simulink model "BD_PRIUS_JPN"  (Simulink 7.9)
settings: Solver=ode1  SolverMode=SingleTasking  StartTime=0.0  StopTime=max(cyc_mph(:,1))  FixedStep=1  MaxStep=1  RelTol=1e-3  AbsTol=1e-3
undefined symbols (not defined in the file): ex_calc, fc_emis
libraries: lib_wheel x2, lib_help x2, lib_transmission x2, lib_electric_machine x2, lib_outputs x1, lib_controls x1, lib_interactive x1, lib_drive_cycle x1, lib_energy_storage x1, lib_exhaust x1, lib_fuel_converter x1, lib_power_bus x1
settings Model: Creator=mokeefe  LastModifiedBy=mokeefe  ExtModeTrigMode=oneshot  ExtModeArmWhenConnect=off
settings Model: ModifiedComment=|
  | mokeefe -- Fri Apr 06 09:40:25 2012 -- Version 1.42
  | Update library links.
settings Model: ModifiedHistory=|
  | mokeefe -- Fri Apr 06 09:40:25 2012 -- Version 1.42
  | Update library links.
  | 
  | mokeefe -- Fri Apr 06 09:31:50 2012 -- Version 1.41
  | Save as latest simulink version.
  | 
  | ssprik -- Wed Sep 24 15:15:04 2003 -- Version 1.40
  | 
  | 
  | abrooker -- Tue May 14 11:47:35 2002 -- Version 1.39
  | 
  | 
  | mokeefe -- Thu Apr 18 08:05:37 2002 -- Version 1.38
  | saving the model:
  | o "without the model browser open"
  | o with only top-level screen visible
  | o and with "fit to view" enabled
settings DataIOCC: LimitDataPoints=off  SaveOutput=off  SaveTime=off
settings OptimizationCC: BooleanDataType=off
settings DebuggingCC: SaveWithParameterizedLinksMsg=none  SignalResolutionControl=TryResolveAllWithWarning  SolverPrmCheckMsg=none  MultiTaskDSMMsg=warning  MultiTaskCondExecSysMsg=none  UnconnectedLineMsg=none  StrictBusMsg=None
settings HardwareCC: TargetUnknown=on
settings RTWCC: TemplateMakefile=grt_vc.tmf  IncludeERTFirstTime=on
settings GRTTargetCC: CombineOutputUpdateFcns=off  GRTInterface=on

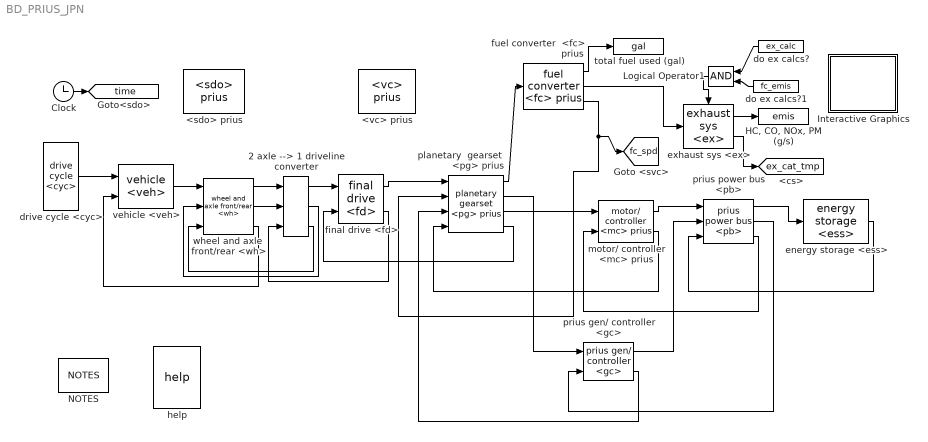
== system BD_PRIUS_JPN ==
  2 axle --> 1 driveline converter : lib_wheel/2 axle --> 1 driveline converter
  <sdo> prius : lib_outputs/<sdo> prius  SystemSampleTime=-1
  <vc> prius : lib_controls/<vc> prius  SystemSampleTime=-1
      link override config traction control: BlockChoice=traction control 2 axle
  Clock : Clock
  "HC, CO, NOx, PM (g/s)" : ToWorkspace  VariableName=emis
      settings: MaxDataPoints=100000
  Interactive Graphics : Subsystem  BlockChoice=off
      settings: AttributesFormatString=%<BlockChoice>  TemplateBlock=lib_interactive/Interactive Graphics  MemberBlocks=off,on
  Logical Operator1 : Logic
  NOTES : lib_help/NOTES  SystemSampleTime=-1
  do ex calcs? : Constant  Value=ex_calc
  do ex calcs?1 : Constant  Value=fc_emis
  drive cycle <cyc> : lib_drive_cycle/drive cycle <cyc>  SystemSampleTime=-1
  energy storage <ess> : lib_energy_storage/energy storage <ess>  SystemSampleTime=-1
      link override ess config: BlockChoice=energy storage <ess>
  exhaust sys <ex> : lib_exhaust/exhaust sys <ex>  SystemSampleTime=-1
  final drive <fd> : lib_transmission/final drive <fd>  SystemSampleTime=-1
  fuel converter  <fc> prius : lib_fuel_converter/fuel converter  <fc> prius  SystemSampleTime=-1
      link override fuel use and EO emis Configurable Subsystem: BlockChoice=fuel use and EO emis
  help : lib_help/help  SystemSampleTime=-1
  motor/ controller <mc> prius : lib_electric_machine/motor// controller <mc> prius  SystemSampleTime=-1
  planetary  gearset  <pg> prius : lib_transmission/planetary  gearset  <pg> prius  SystemSampleTime=-1
  prius gen/ controller <gc> : lib_electric_machine/prius gen// controller <gc>  SystemSampleTime=-1
  prius power bus <pb> : lib_power_bus/prius power bus <pb>  SystemSampleTime=-1
  total fuel used (gal) : ToWorkspace  VariableName=gal
      settings: MaxDataPoints=50000
  vehicle <veh> : lib_vehicle/vehicle <veh>  SystemSampleTime=-1
      link override record achieved force outputs/rolling resistance force: BlockChoice=force req'd to overcome rolling resistance (N)
      link override rolling resistance force: BlockChoice=force req'd to overcome rolling resistance (N)
      link override vehicle speed: BlockChoice=vehicle speed (m/s)
  wheel and axle  front/rear <wh> : lib_wheel/wheel and axle  front//rear <wh>  SystemSampleTime=-1
  tag scope: ex_cat_tmp=global, fc_spd=global, time=global
  wires:
  drive cycle <cyc>/1 -> vehicle <veh>/1
  Clock/1 -> [time]
  Logical Operator1/1 -> exhaust sys <ex>/Enable
  final drive <fd>/1 -> planetary  gearset  <pg> prius/1
  planetary  gearset  <pg> prius/4 -> final drive <fd>/2
  planetary  gearset  <pg> prius/3 -> motor/ controller <mc> prius/1
  planetary  gearset  <pg> prius/1 -> fuel converter  <fc> prius/1
  prius power bus <pb>/1 -> energy storage <ess>/1
  energy storage <ess>/1 -> prius power bus <pb>/3
  motor/ controller <mc> prius/2 -> planetary  gearset  <pg> prius/4
  planetary  gearset  <pg> prius/2 -> prius gen/ controller <gc>/1
  prius gen/ controller <gc>/2 -> planetary  gearset  <pg> prius/3
  motor/ controller <mc> prius/1 -> prius power bus <pb>/1
  prius power bus <pb>/3 -> motor/ controller <mc> prius/2
  prius gen/ controller <gc>/1 -> prius power bus <pb>/2
  prius power bus <pb>/2 -> prius gen/ controller <gc>/2
  fuel converter  <fc> prius/2 -> exhaust sys <ex>/1
  fuel converter  <fc> prius/1 -> total fuel used (gal)/1
  fuel converter  <fc> prius/3 -> planetary  gearset  <pg> prius/2, [fc_spd]
  do ex calcs?/1 -> Logical Operator1/1
  exhaust sys <ex>/1 -> "HC, CO, NOx, PM (g/s)"/1
  do ex calcs?1/1 -> Logical Operator1/2
  exhaust sys <ex>/2 -> [ex_cat_tmp]
  vehicle <veh>/1 -> wheel and axle  front/rear <wh>/1
  wheel and axle  front/rear <wh>/1 -> 2 axle --> 1 driveline converter/1
  wheel and axle  front/rear <wh>/2 -> 2 axle --> 1 driveline converter/2
  2 axle --> 1 driveline converter/1 -> final drive <fd>/1
  2 axle --> 1 driveline converter/2 -> wheel and axle  front/rear <wh>/2
  2 axle --> 1 driveline converter/3 -> wheel and axle  front/rear <wh>/3
  final drive <fd>/2 -> 2 axle --> 1 driveline converter/3
  wheel and axle  front/rear <wh>/3 -> vehicle <veh>/2

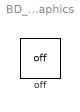
== system BD_PRIUS_JPN/Interactive Graphics ==
  off : lib_interactive/off  Tag=Altia_off  SystemSampleTime=-1
